simulink model "experiment"  (R2020a)
settings: Solver=VariableStepAuto  StartTime=0.0  StopTime=100  RelTol=1e-3
settings Model: Creator=pyz  LastModifiedBy=Wesley
settings DataIOCC: ReturnWorkspaceOutputs=off
settings DebuggingCC: ArithmeticOperatorsInVariantConditions=warning
settings SFSimCC: SimUseLocalCustomCode=off  CustomCodeUndefinedFunction=UseInterfaceOnly
settings RTWCC: RTWUseLocalCustomCode=off

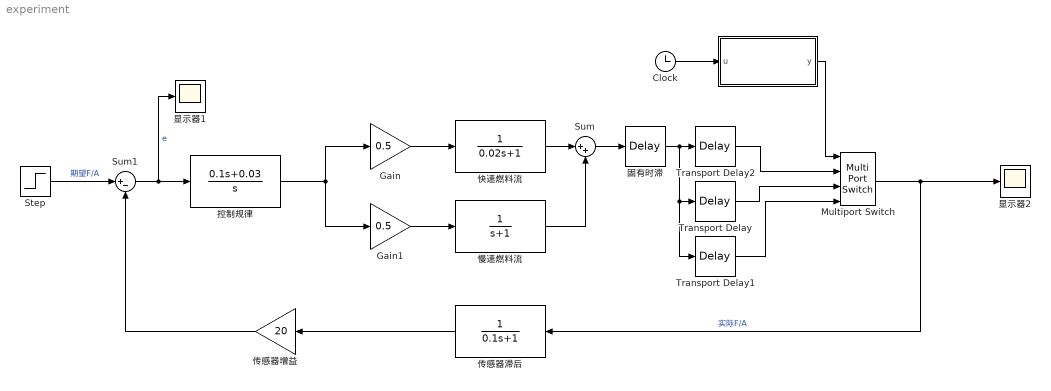
== system experiment ==
  " " : MATLAB Function  TreatAsAtomicUnit=on
  Clock : Clock
      settings: Decimation=200
  Gain : Gain  Gain=0.5
  Gain1 : Gain  Gain=0.5
  Multiport Switch : MultiPortSwitch
  Step : Step  Time=0  After=0.018  SampleTime=0
  Sum : Sum  Inputs=|++
  Sum1 : Sum  Inputs=|+-
  Transport Delay : TransportDelay  DelayTime=0.06
  Transport Delay1 : TransportDelay  DelayTime=0.04
  Transport Delay2 : TransportDelay  DelayTime=0.12
  传感器增益 : Gain  Gain=20
  传感器滞后 : TransferFcn  Denominator=[0.1 1]
  固有时滞 : TransportDelay  DelayTime=0.1
  快速燃料流 : TransferFcn  Denominator=[0.02 1]
  慢速燃料流 : TransferFcn  Denominator=[1 1]
  控制规律 : TransferFcn  Numerator=[0.1 0.03]  Denominator=[1 0]
  显示器1 : Scope
  显示器2 : Scope
  wires:
  Gain/1 -> 快速燃料流/1
  Gain1/1 -> 慢速燃料流/1
  快速燃料流/1 -> Sum/1
  慢速燃料流/1 -> Sum/2
  控制规律/1 -> Gain/1, Gain1/1
  Sum1/1 -> 显示器1/1, 控制规律/1  "e"
  Multiport Switch/1 -> 显示器2/1, 传感器滞后/1  "实际F/A"
  传感器滞后/1 -> 传感器增益/1
  Step/1 -> Sum1/1  "期望F/A"
  传感器增益/1 -> Sum1/2
  " "/1(y) -> Multiport Switch/1
  Sum/1 -> 固有时滞/1
  Transport Delay2/1 -> Multiport Switch/2
  Transport Delay/1 -> Multiport Switch/3
  Clock/1 -> " "/1(u)
  Transport Delay1/1 -> Multiport Switch/4
  固有时滞/1 -> Transport Delay2/1, Transport Delay1/1, Transport Delay/1

== matlab function experiment/  ==
  data: u input; y output
function y = fas(u)
if u>30&&u<60
    y=2;
elseif u>60
    y=3;
else
    y=1;
end
end
